simulink model "untitled"  (R2016a)
settings: Solver=VariableStepAuto  StartTime=0.0  StopTime=10.0  RelTol=1e-3
settings Model: Creator=Gianluigi  LastModifiedBy=Gianluigi

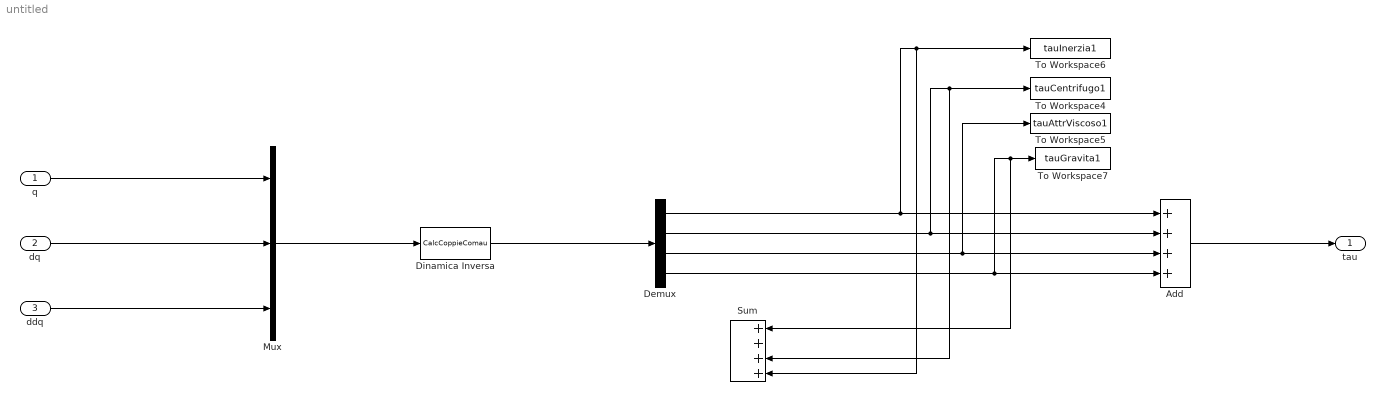
== system untitled ==
  q : Inport
  dq : Inport  Port=2
  ddq : Inport  Port=3
  Add : Sum  Inputs=++++
  Demux : Demux
  Dinamica Inversa : MATLABFcn  MATLABFcn=CalcCoppieComau  OutputDimensions=24
  Mux : Mux  Inputs=3
  Sum : Sum  Inputs=++++
  To Workspace4 : ToWorkspace  VariableName=tauCentrifugo1  SampleTime=-1
  To Workspace5 : ToWorkspace  VariableName=tauAttrViscoso1  SampleTime=-1
  To Workspace6 : ToWorkspace  VariableName=tauInerzia1  SampleTime=-1
  To Workspace7 : ToWorkspace  VariableName=tauGravita1  SampleTime=-1
  tau : Outport
  wires:
  q/1 -> Mux/1
  Mux/1 -> Dinamica Inversa/1
  dq/1 -> Mux/2
  ddq/1 -> Mux/3
  Dinamica Inversa/1 -> Demux/1
  Add/1 -> tau/1
  Demux/1 -> Add/1, Sum/4, To Workspace6/1
  Demux/2 -> Add/2, To Workspace4/1, Sum/3
  Demux/3 -> Add/3, To Workspace5/1
  Demux/4 -> Add/4, To Workspace7/1, Sum/1
